simulink model "sim_part3"  (R2020a)
settings: Solver=VariableStepAuto  StartTime=0.0  StopTime=10.0  RelTol=1e-3
values from neighbouring files (symbols this model uses):
  b_s = 0.28    [part1.m]    (also in part2.m; part3.m; stability_plot.m)
  f_s = 0.2    [part1.m]    (also in part2.m; part3.m; stability_plot.m)
  g_s = 0.5    [part1.m]    (also in part2.m; part3.m; stability_plot.m)
  i_b_m = 0.025    [part1.m]    (also in part2.m; part3.m; stability_plot.m)
  i_cb = 0.1    [part1.m]    (also in part2.m; part3.m; stability_plot.m)
  I_eps = 0.1    [part1.m]    (also in part2.m; part3.m; stability_plot.m)
  i_f_m = 0.05    [part1.m]    (also in part2.m; part3.m; stability_plot.m)
  K_0 = 0.08    [part1.m]    (also in part2.m; part3.m; stability_plot.m)
  K_p = 15    [part1.m]    (also in part2.m; part3.m; stability_plot.m)
  lambda = 0.002    [part1.m]    (also in part2.m; part3.m; stability_plot.m)
  lambda_f = 0.005    [part1.m]    (also in part2.m; part3.m; stability_plot.m)
  loss_eq = 2    [part1.m]    (also in part2.m; part3.m; stability_plot.m)
  R = 1    [part1.m]    (also in part2.m; part3.m; stability_plot.m)
  r_b = 0.1    [part1.m]    (also in part2.m; part3.m; stability_plot.m)
  r_f = 0.1    [part1.m]    (also in part2.m; part3.m; stability_plot.m)
  r_g = 0.1    [part1.m]    (also in part2.m; part3.m; stability_plot.m)
  T_f = 0.5    [part1.m]    (also in part2.m; part3.m; stability_plot.m)
  T_g = 1    [part1.m]    (also in part2.m; part3.m; stability_plot.m)
  T_h = 0.1    [part1.m]    (also in part2.m; part3.m; stability_plot.m)
  T_i = 8    [part1.m]    (also in part2.m; part3.m; stability_plot.m)
  T_k = 0.1    [part1.m]    (also in part2.m; part3.m; stability_plot.m)
  t_x = 0.3    [part1.m]    (also in part2.m; part3.m; stability_plot.m)
settings Model: Creator=erlended  LastModifiedBy=erlended

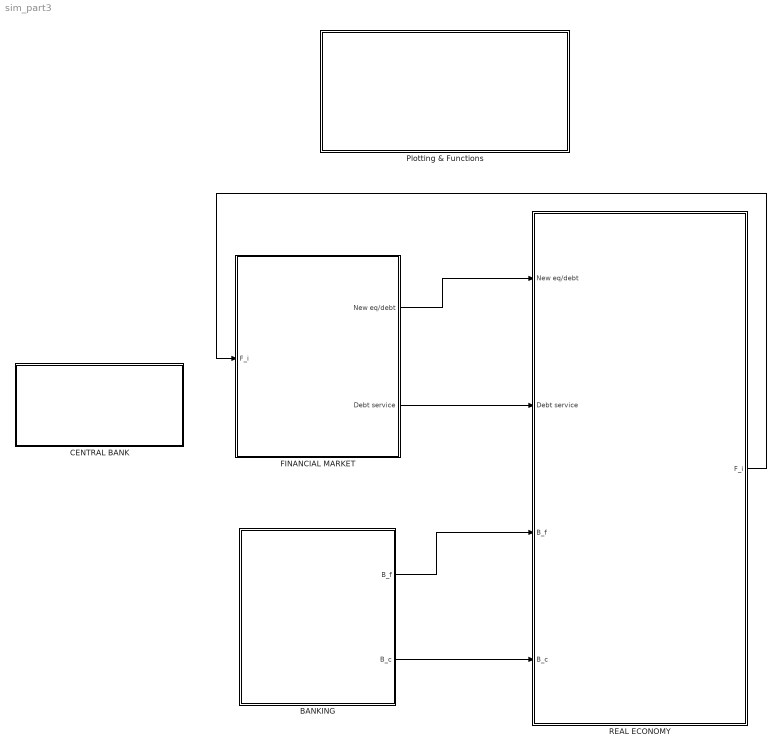
== system sim_part3 ==
  BANKING : Subsystem
  CENTRAL BANK : Subsystem
  FINANCIAL MARKET : Subsystem
  Plotting & Functions : Subsystem
  REAL ECONOMY : Subsystem
  wires:
  BANKING/1(B_f) -> REAL ECONOMY/3(B_f)
  BANKING/2(B_c) -> REAL ECONOMY/4(B_c)
  FINANCIAL MARKET/1(New eq/debt) -> REAL ECONOMY/1(New eq/debt)
  FINANCIAL MARKET/2(Debt service) -> REAL ECONOMY/2(Debt service)
  REAL ECONOMY/1(F_i) -> FINANCIAL MARKET/1(F_i)

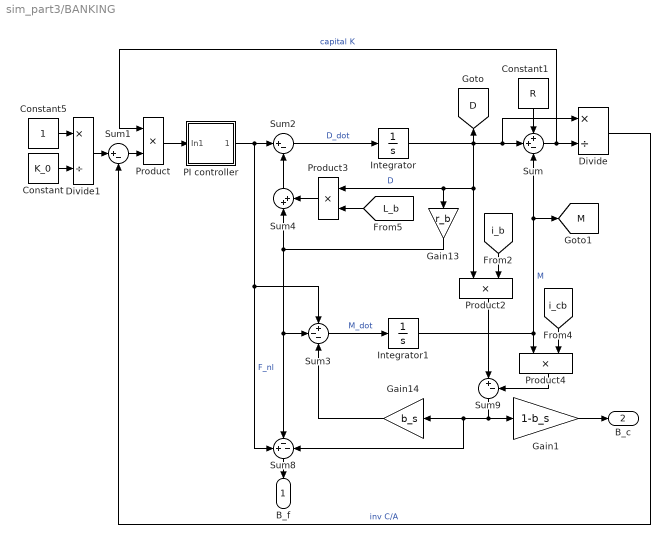
== system sim_part3/BANKING ==
  Constant : Constant  Value=K_0
  Constant1 : Constant  Value=R
  Constant5 : Constant
  Divide : Product  Inputs=*/
  Divide1 : Product  Inputs=*/
  Gain1 : Gain  Gain=1-b_s
  Gain13 : Gain  Gain=r_b
  Gain14 : Gain  Gain=b_s
  Integrator : Integrator
  Integrator1 : Integrator
  PI controller : Subsystem
  Product{,2..4} (4 alike) : Product
  Sum : Sum  Inputs=++-
  Sum1 : Sum  Inputs=|+-
  Sum2 : Sum  Inputs=|+-
  Sum3 : Sum  Inputs=+--
  Sum4 : Sum  Inputs=|++
  Sum8 : Sum  Inputs=+--
  Sum9 : Sum  Inputs=|+-
  B_f : Outport
  B_c : Outport  Port=2
  tag scope: D=global, M=global
  wires:
  Integrator/1 -> [D], Product3/1, Gain13/1, Product2/1, Sum/2, Divide/1  "D"
  Integrator1/1 -> Product4/1, [M], Sum/3  "M"
  Sum/1 -> Divide/2, Product/1  "capital K"
  Sum4/1 -> Sum2/2
  Gain13/1 -> Sum8/2, Sum3/2, Sum4/1
  Sum9/1 -> Gain14/1, Sum8/3, Gain1/1
  Sum2/1 -> Integrator/1  "D_dot"
  Constant1/1 -> Sum/1
  Divide/1 -> Sum1/2  "inv C/A"
  Sum1/1 -> Product/2
  Sum3/1 -> Integrator1/1  "M_dot"
  Product2/1 -> Sum9/1
  Product4/1 -> Sum9/2
  Constant5/1 -> Divide1/1
  Divide1/1 -> Sum1/1
  Gain14/1 -> Sum3/3
  Constant/1 -> Divide1/2
  [i_b] -> Product2/2
  [i_cb] -> Product4/2
  [L_b] -> Product3/2
  Product3/1 -> Sum4/2
  PI controller/1(Out1) -> Sum2/1, Sum8/1, Sum3/1  "F_nl"
  Product/1 -> PI controller/1(In1)
  Gain1/1 -> B_c/1
  Sum8/1 -> B_f/1

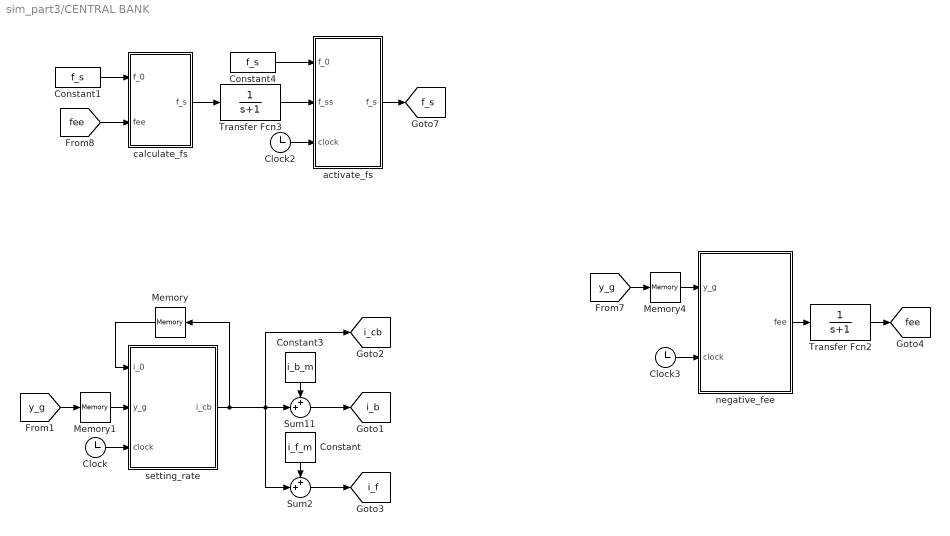
== system sim_part3/CENTRAL BANK ==
  Clock : Clock
  Clock2 : Clock
  Clock3 : Clock
  Constant : Constant  Value=i_f_m
  Constant1 : Constant  Value=f_s
  Constant3 : Constant  Value=i_b_m
  Constant4 : Constant  Value=f_s
  Memory : Memory  InitialCondition=i_cb
  Memory1 : Memory
  Memory4 : Memory
  Sum11 : Sum  Inputs=++|
  Sum2 : Sum  Inputs=++|
  Transfer Fcn2 : TransferFcn  Denominator=[1 1]
  Transfer Fcn3 : TransferFcn  Denominator=[1 1]
  activate_fs : MATLAB Function  TreatAsAtomicUnit=on
  calculate_fs : MATLAB Function  TreatAsAtomicUnit=on
  negative_fee : MATLAB Function  TreatAsAtomicUnit=on
  setting_rate : MATLAB Function  TreatAsAtomicUnit=on
  tag scope: f_s=global, fee=global, i_b=global, i_cb=global, i_f=global
  wires:
  Constant/1 -> Sum2/1
  setting_rate/1(i_cb) -> Memory/1, [i_cb], Sum11/2, Sum2/2
  Constant3/1 -> Sum11/1
  Sum11/1 -> [i_b]
  [y_g] -> Memory1/1
  Memory/1 -> setting_rate/1(i_0)
  Clock/1 -> setting_rate/3(clock)
  Memory1/1 -> setting_rate/2(y_g)
  Sum2/1 -> [i_f]
  Clock2/1 -> activate_fs/3(clock)
  [fee] -> calculate_fs/2(fee)
  Constant4/1 -> activate_fs/1(f_0)
  Transfer Fcn3/1 -> activate_fs/2(f_ss)
  Clock3/1 -> negative_fee/2(clock)
  Constant1/1 -> calculate_fs/1(f_0)
  Memory4/1 -> negative_fee/1(y_g)
  [y_g] -> Memory4/1
  negative_fee/1(fee) -> Transfer Fcn2/1
  Transfer Fcn2/1 -> [fee]
  activate_fs/1(f_s) -> [f_s]
  calculate_fs/1(f_s) -> Transfer Fcn3/1

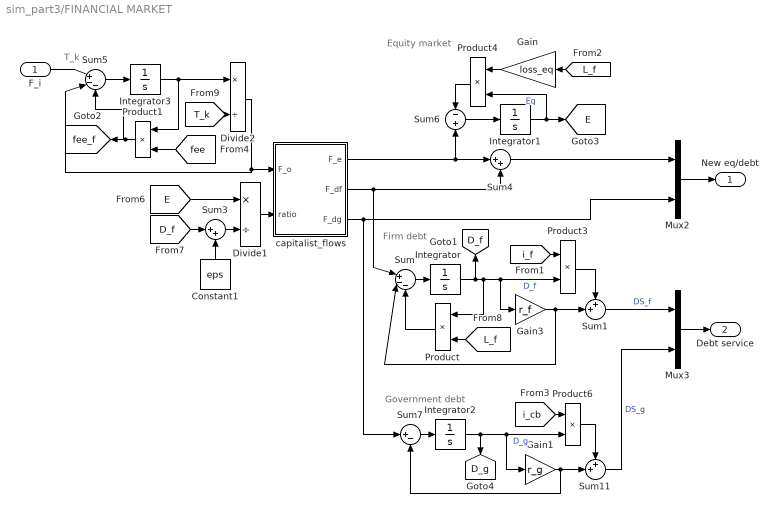
== system sim_part3/FINANCIAL MARKET ==
  note: Firm debt
  note: T_k
  note: Government debt
  note: Equity market
  F_i : Inport
  Constant1 : Constant  Value=eps
  Divide1 : Product  Inputs=*/
  Divide2 : Product  Inputs=*/
  Gain : Gain  Gain=loss_eq
  Gain1 : Gain  Gain=r_g
  Gain3 : Gain  Gain=r_f
  Integrator{,1..3} (4 alike) : Integrator
  Mux2 : Mux  Inputs=2
  Mux3 : Mux  Inputs=2
  Product{,1,3..4,6} (5 alike) : Product
  Sum : Sum  Inputs=|+--
  Sum1 : Sum  Inputs=++|
  Sum11 : Sum  Inputs=++|
  Sum3 : Sum  Inputs=|++
  Sum4 : Sum  Inputs=|++
  Sum5 : Sum  Inputs=|+--
  Sum6 : Sum  Inputs=-+
  Sum7 : Sum  Inputs=|+-
  capitalist_flows : MATLAB Function  TreatAsAtomicUnit=on
  New eq/debt : Outport
  Debt service : Outport  Port=2
  tag scope: D_f=global, D_g=global, E=global, fee_f=global
  wires:
  Mux3/1 -> Debt service/1
  F_i/1 -> Sum5/1
  Gain/1 -> Product4/1
  capitalist_flows/1(F_e) -> Sum6/2, Sum4/1
  Sum5/1 -> Integrator3/1
  Sum1/1 -> Mux3/1  "DS_f"
  Integrator/1 -> [D_f], Gain3/1, Product3/2, Product/1  "D_f"
  Integrator3/1 -> Product1/1, Divide2/1
  [i_f] -> Product3/1
  Sum11/1 -> Mux3/2  "DS_g"
  Product3/1 -> Sum1/1
  [L_f] -> Product/2
  [L_f] -> Gain/1
  Sum/1 -> Integrator/1
  Divide2/1 -> capitalist_flows/1(F_o), Sum5/2
  [E] -> Divide1/1
  Product4/1 -> Sum6/1
  Gain1/1 -> Sum11/2, Sum7/2
  Product/1 -> Sum/3
  [D_f] -> Sum3/1
  Sum6/1 -> Integrator1/1
  Constant1/1 -> Sum3/2
  capitalist_flows/2(F_df) -> Sum4/2, Sum/1
  Product6/1 -> Sum11/1
  Sum3/1 -> Divide1/2
  Divide1/1 -> capitalist_flows/2(ratio)
  Sum4/1 -> Mux2/1
  Integrator1/1 -> [E], Product4/2  "Eq"
  Mux2/1 -> New eq/debt/1
  [T_k] -> Divide2/2
  Sum7/1 -> Integrator2/1
  Gain3/1 -> Sum1/2, Sum/2
  Integrator2/1 -> [D_g], Product6/2, Gain1/1  "D_g"
  [i_cb] -> Product6/1
  capitalist_flows/3(F_dg) -> Mux2/2, Sum7/1
  [fee] -> Product1/2
  Product1/1 -> Sum5/3, [fee_f]

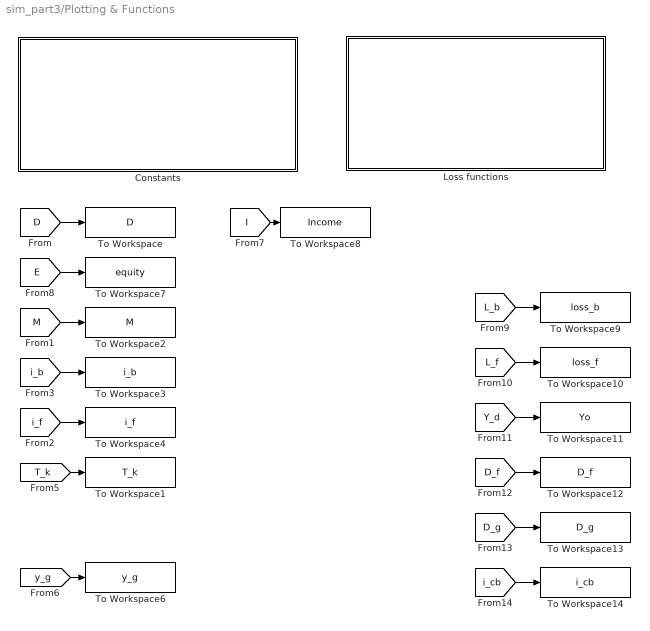
== system sim_part3/Plotting & Functions ==
  Constants : Subsystem
  Loss functions : Subsystem
  To Workspace : ToWorkspace  VariableName=D  SaveFormat=Timeseries  SampleTime=-1
  To Workspace1 : ToWorkspace  VariableName=T_k  SaveFormat=Timeseries  SampleTime=-1
  To Workspace10 : ToWorkspace  VariableName=loss_f  SaveFormat=Timeseries  SampleTime=-1
  To Workspace11 : ToWorkspace  VariableName=Yo  SaveFormat=Timeseries  SampleTime=-1
  To Workspace12 : ToWorkspace  VariableName=D_f  SaveFormat=Timeseries  SampleTime=-1
  To Workspace13 : ToWorkspace  VariableName=D_g  SaveFormat=Timeseries  SampleTime=-1
  To Workspace14 : ToWorkspace  VariableName=i_cb  SaveFormat=Timeseries  SampleTime=-1
  To Workspace2 : ToWorkspace  VariableName=M  SaveFormat=Timeseries  SampleTime=-1
  To Workspace3 : ToWorkspace  VariableName=i_b  SaveFormat=Timeseries  SampleTime=-1
  To Workspace4 : ToWorkspace  VariableName=i_f  SaveFormat=Timeseries  SampleTime=-1
  To Workspace6 : ToWorkspace  VariableName=y_g  SaveFormat=Timeseries  SampleTime=-1
  To Workspace7 : ToWorkspace  VariableName=equity  SaveFormat=Timeseries  SampleTime=-1
  To Workspace8 : ToWorkspace  VariableName=Income  SaveFormat=Timeseries  SampleTime=-1
  To Workspace9 : ToWorkspace  VariableName=loss_b  SaveFormat=Timeseries  SampleTime=-1
  wires:
  [D] -> To Workspace/1
  [E] -> To Workspace7/1
  [M] -> To Workspace2/1
  [i_b] -> To Workspace3/1
  [i_f] -> To Workspace4/1
  [T_k] -> To Workspace1/1
  [y_g] -> To Workspace6/1
  [I] -> To Workspace8/1
  [L_b] -> To Workspace9/1
  [L_f] -> To Workspace10/1
  [Y_d] -> To Workspace11/1
  [D_f] -> To Workspace12/1
  [D_g] -> To Workspace13/1
  [i_cb] -> To Workspace14/1

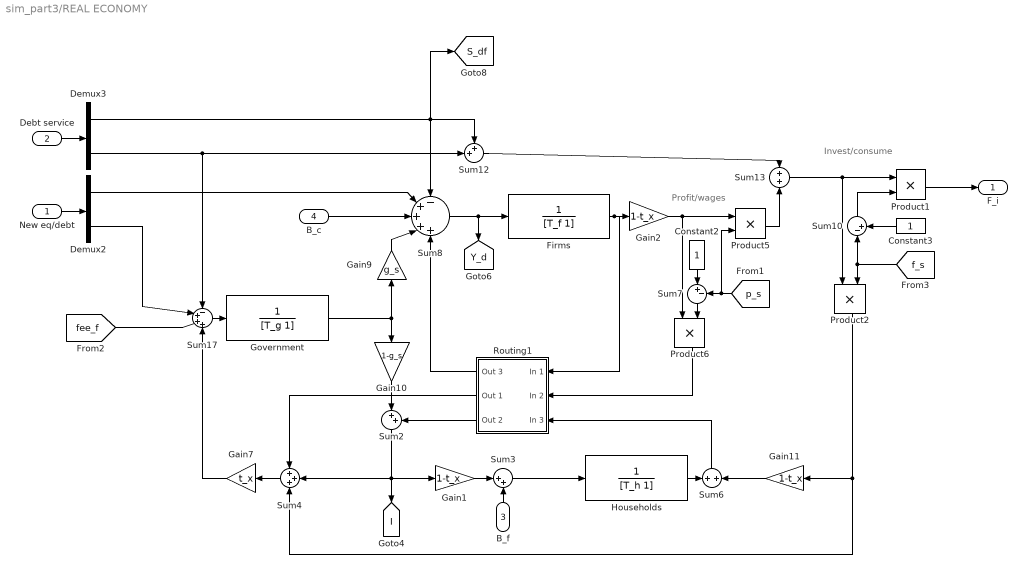
== system sim_part3/REAL ECONOMY ==
  note: Invest/consume
  note: Profit/wages
  New eq/debt : Inport
  Debt service : Inport  Port=2
  B_f : Inport  Port=3
  B_c : Inport  Port=4
  Constant2 : Constant
  Constant3 : Constant
  Demux2 : Demux  Outputs=2
  Demux3 : Demux  Outputs=2
  Firms : TransferFcn  Denominator=[T_f 1]
  Gain1 : Gain  Gain=1-t_x
  Gain10 : Gain  Gain=1-g_s
  Gain11 : Gain  Gain=1-t_x
  Gain2 : Gain  Gain=1-t_x
  Gain7 : Gain  Gain=t_x
  Gain9 : Gain  Gain=g_s
  Government : TransferFcn  Denominator=[T_g 1]
  Households : TransferFcn  Denominator=[T_h 1]
  Product{1..2,5..6} (4 alike) : Product
  Routing1 : Subsystem
  Sum10 : Sum  Inputs=|-+
  Sum12 : Sum  Inputs=++|
  Sum13 : Sum
  Sum17 : Sum  Inputs=-+++
  Sum2 : Sum  Inputs=|++
  Sum3 : Sum  Inputs=|++
  Sum4 : Sum  Inputs=+++
  Sum6 : Sum  Inputs=+|+
  Sum7 : Sum  Inputs=|+-
  Sum8 : Sum  Inputs=-++++
  F_i : Outport
  tag scope: I=global, S_df=global, Y_d=global
  wires:
  Debt service/1 -> Demux3/1
  New eq/debt/1 -> Demux2/1
  Product2/1 -> Gain11/1, Sum4/3
  Sum12/1 -> Sum13/1
  Sum4/1 -> Gain7/1
  B_f/1 -> Sum3/2
  Firms/1 -> Routing1/1(In 1), Gain2/1
  Constant2/1 -> Sum7/1
  Sum13/1 -> Product2/1, Product1/1
  [f_s] -> Sum10/1, Product2/2
  Gain1/1 -> Sum3/1
  Sum2/1 -> Sum4/2, [I], Gain1/1
  Sum3/1 -> Households/1
  Gain2/1 -> Product5/1, Product6/1
  B_c/1 -> Sum8/3
  Sum10/1 -> Product1/2
  Gain10/1 -> Sum2/1
  Demux2/1 -> Sum8/2
  Sum8/1 -> [Y_d], Firms/1
  Sum17/1 -> Government/1
  Gain11/1 -> Sum6/2
  Sum7/1 -> Product6/2
  Sum6/1 -> Routing1/3(In 3)
  Demux3/2 -> Sum12/2, Sum17/1
  Routing1/2(Out 1) -> Sum4/1
  Product6/1 -> Routing1/2(In 2)
  Demux3/1 -> [S_df], Sum12/1, Sum8/1
  Government/1 -> Gain9/1, Gain10/1
  Gain9/1 -> Sum8/4
  Households/1 -> Sum6/1
  Product5/1 -> Sum13/2
  Routing1/3(Out 2) -> Sum2/2
  Routing1/1(Out 3) -> Sum8/5
  Constant3/1 -> Sum10/2
  Demux2/2 -> Sum17/2
  Product1/1 -> F_i/1
  Gain7/1 -> Sum17/4
  [p_s] -> Sum7/2, Product5/2
  [fee_f] -> Sum17/3

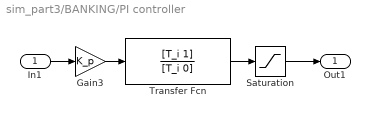
== system sim_part3/BANKING/PI controller ==
  In1 : Inport
  Gain3 : Gain  Gain=K_p
  Saturation : Saturate  UpperLimit=1000  LowerLimit=0
  Transfer Fcn : TransferFcn  Numerator=[T_i 1]  Denominator=[T_i 0]
  Out1 : Outport
  wires:
  Gain3/1 -> Transfer Fcn/1
  Transfer Fcn/1 -> Saturation/1
  In1/1 -> Gain3/1
  Saturation/1 -> Out1/1

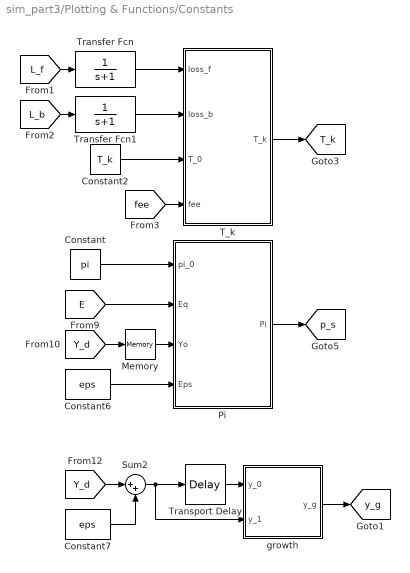
== system sim_part3/Plotting & Functions/Constants ==
  Constant : Constant  Value=pi
  Constant2 : Constant  Value=T_k
  Constant6 : Constant  Value=eps
  Constant7 : Constant  Value=eps
  Memory : Memory
  Pi : MATLAB Function  TreatAsAtomicUnit=on
  Sum2 : Sum  Inputs=|++
  T_k : MATLAB Function  TreatAsAtomicUnit=on
  Transfer Fcn : TransferFcn  Denominator=[1 1]
  Transfer Fcn1 : TransferFcn  Denominator=[1 1]
  Transport Delay : TransportDelay
  growth : MATLAB Function  TreatAsAtomicUnit=on
  tag scope: T_k=global, p_s=global, y_g=global
  wires:
  Pi/1(Pi) -> [p_s]
  [E] -> Pi/2(Eq)
  Memory/1 -> Pi/3(Yo)
  Constant/1 -> Pi/1(pi_0)
  [Y_d] -> Memory/1
  Constant2/1 -> T_k/3(T_0)
  Constant6/1 -> Pi/4(Eps)
  Transfer Fcn/1 -> T_k/1(loss_f)
  [L_f] -> Transfer Fcn/1
  [L_b] -> Transfer Fcn1/1
  Transfer Fcn1/1 -> T_k/2(loss_b)
  Sum2/1 -> Transport Delay/1, growth/2(y_1)
  Transport Delay/1 -> growth/1(y_0)
  Constant7/1 -> Sum2/2
  [Y_d] -> Sum2/1
  growth/1(y_g) -> [y_g]
  [fee] -> T_k/4(fee)
  T_k/1(T_k) -> [T_k]

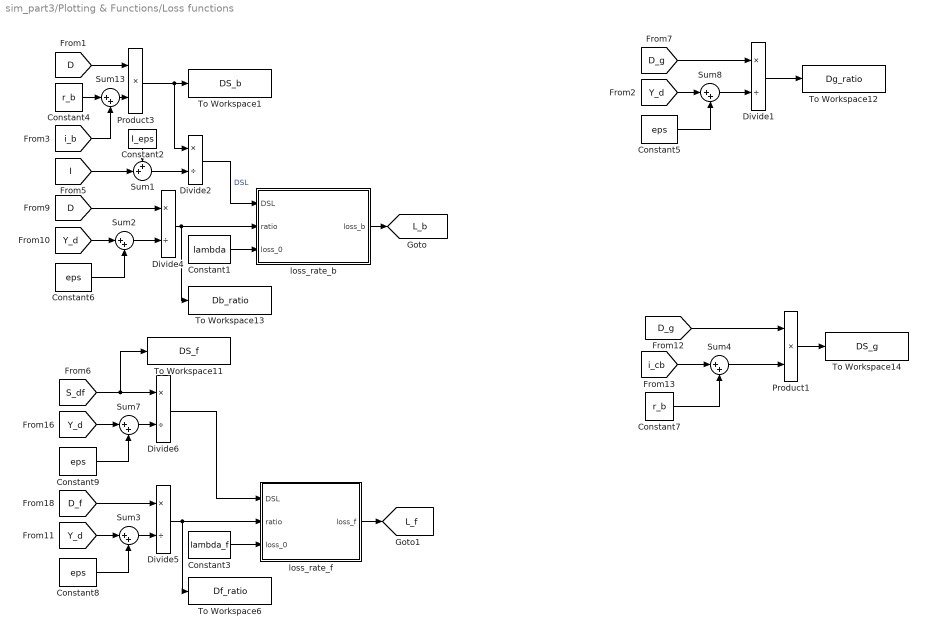
== system sim_part3/Plotting & Functions/Loss functions ==
  Constant1 : Constant  Value=lambda
  Constant2 : Constant  Value=I_eps
  Constant3 : Constant  Value=lambda_f
  Constant4 : Constant  Value=r_b
  Constant{5..6,8..9} (4 alike) : Constant  Value=eps
  Constant7 : Constant  Value=r_b
  Divide{1..2,4..6} (5 alike) : Product  Inputs=*/
  Product1 : Product
  Product3 : Product
  Sum1 : Sum  Inputs=++|
  Sum{2..4,7..8,13} (6 alike) : Sum  Inputs=|++
  To Workspace1 : ToWorkspace  VariableName=DS_b  SaveFormat=Timeseries  SampleTime=-1
  To Workspace11 : ToWorkspace  VariableName=DS_f  SaveFormat=Timeseries  SampleTime=-1
  To Workspace12 : ToWorkspace  VariableName=Dg_ratio  SaveFormat=Timeseries  SampleTime=-1
  To Workspace13 : ToWorkspace  VariableName=Db_ratio  SaveFormat=Timeseries  SampleTime=-1
  To Workspace14 : ToWorkspace  VariableName=DS_g  SaveFormat=Timeseries  SampleTime=-1
  To Workspace6 : ToWorkspace  VariableName=Df_ratio  SaveFormat=Timeseries  SampleTime=-1
  loss_rate_b : MATLAB Function  TreatAsAtomicUnit=on
  loss_rate_f : MATLAB Function  TreatAsAtomicUnit=on
  tag scope: L_b=global, L_f=global
  wires:
  Constant1/1 -> loss_rate_b/3(loss_0)
  Constant4/1 -> Sum13/1
  Product3/1 -> Divide2/1, To Workspace1/1
  [D] -> Product3/1
  [i_b] -> Sum13/2
  loss_rate_b/1(loss_b) -> [L_b]
  Sum13/1 -> Product3/2
  Divide5/1 -> To Workspace6/1, loss_rate_f/2(ratio)
  loss_rate_f/1(loss_f) -> [L_f]
  Constant3/1 -> loss_rate_f/3(loss_0)
  Divide1/1 -> To Workspace12/1
  Sum2/1 -> Divide4/2
  [D] -> Divide4/1
  Divide4/1 -> To Workspace13/1, loss_rate_b/2(ratio)
  Divide2/1 -> loss_rate_b/1(DSL)  "DSL"
  Divide6/1 -> loss_rate_f/1(DSL)
  Sum4/1 -> Product1/2
  Product1/1 -> To Workspace14/1
  [D_g] -> Product1/1
  [Y_d] -> Sum2/1
  Constant6/1 -> Sum2/2
  Constant9/1 -> Sum7/2
  [Y_d] -> Sum7/1
  Sum7/1 -> Divide6/2
  [S_df] -> To Workspace11/1, Divide6/1
  Constant8/1 -> Sum3/2
  [Y_d] -> Sum3/1
  Sum3/1 -> Divide5/2
  [D_f] -> Divide5/1
  Sum8/1 -> Divide1/2
  [Y_d] -> Sum8/1
  Constant5/1 -> Sum8/2
  [D_g] -> Divide1/1
  [i_cb] -> Sum4/1
  Constant7/1 -> Sum4/2
  Sum1/1 -> Divide2/2
  [I] -> Sum1/2
  Constant2/1 -> Sum1/1

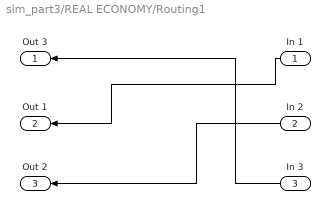
== system sim_part3/REAL ECONOMY/Routing1 ==
  In 1 : Inport
  In 2 : Inport  Port=2
  In 3 : Inport  Port=3
  Out 3 : Outport
  Out 1 : Outport  Port=2
  Out 2 : Outport  Port=3
  wires:
  In 3/1 -> Out 3/1
  In 2/1 -> Out 2/1
  In 1/1 -> Out 1/1

== matlab function sim_part3/Plotting & Functions/Loss functions/loss_rate_b ==
  data: DSL input; ratio input; loss_b output; loss_0 input
function loss_b = fcn(DSL, ratio,loss_0)

loss_b = 0.0025*(ratio/1.6)^6+0.05*DSL^6+loss_0;

== matlab function sim_part3/Plotting & Functions/Loss functions/loss_rate_f ==
  data: DSL input; ratio input; loss_f output; loss_0 input
function loss_f = fcn(DSL, ratio,loss_0)

loss_f = 0.0015*(ratio)^4+(1.5*DSL)^4+loss_0;

== matlab function sim_part3/Plotting & Functions/Constants/T_k ==
  data: loss_f input; loss_b input; T_k output; T_0 input; fee input
function T_k = fcn(loss_f, loss_b, T_0, fee)

T_k = 20*loss_f+60*loss_b+T_0-3*fee;

== matlab function sim_part3/Plotting & Functions/Constants/Pi ==
  data: pi_0 input; Pi output; Eq input; Yo input; Eps input
function Pi = fcn(pi_0, Eq, Yo, Eps)

Pi = 0.05*Eq/(Yo+Eps)+pi_0;
if Pi > 0.6
    Pi = 0.6; 
end

== matlab function sim_part3/Plotting & Functions/Constants/growth ==
  data: y_0 input; y_g output; y_1 input
function y_g = fcn(y_0, y_1)

y_g = (y_1-y_0)/y_0;

== matlab function sim_part3/CENTRAL BANK/setting_rate ==
  data: i_0 input; y_g input; i_cb output; clock input
function i_cb = fcn(i_0, y_g, clock)

i_cb = i_0;

if y_g < 0.01 && clock > 5
    i_cb = i_0 - 0.005;
elseif y_g > 0.06 && clock > 5 
   i_cb = i_0 + 0.0025;
%elseif y_g > 0.04 && clock >= 50
%    i_cb = i_0 + 0.0025;
end

if i_cb <= 0
    i_cb = 0;
end

== matlab function sim_part3/CENTRAL BANK/calculate_fs ==
  data: f_0 input; f_s output; fee input
function f_s = fcn(f_0, fee)

f_s = f_0+15*fee;

== matlab function sim_part3/CENTRAL BANK/negative_fee ==
  data: y_g input; fee output; clock input
function fee = fcn(y_g, clock)
fee = 0; 

%if y_g < 0.01 && clock > 50
%    fee = 0.02;
%elseif  y_g < 0.03 && clock > 50
%    fee = 0.015;  
if  y_g < 0.06 && clock > 50
    fee = 0.01;   
end

%{
if y_g < 0.02 && clock > 50
    fee = 0.02;
elseif  y_g < 0.03 && clock > 50
    fee = 0.015;  
elseif  y_g < 0.04 && clock > 50
    fee = 0.01;   
end
%}

== matlab function sim_part3/CENTRAL BANK/activate_fs ==
  data: f_0 input; f_s output; f_ss input; clock input
function f_s = fcn(f_0, f_ss, clock)
f_s = f_0;
if clock > 50 
    f_s = f_ss; 
end

== matlab function sim_part3/FINANCIAL MARKET/capitalist_flows ==
  data: F_o input; F_e output; F_df output; F_dg output; ratio input
function [F_e,F_df,F_dg]= fcn(F_o, ratio)
F_dg = F_o*0.2;

if ratio > 1
    F_e = F_o*(0.5 - 0.1*ratio);
    F_df = F_o*(0.3 + 0.1*ratio);
else
    F_e = F_o*(0.5 + 0.1*ratio);
    F_df = F_o*(0.3 - 0.1*ratio);
end
